simulink model "LPV_Test"  (R2018a)
settings: Solver=VariableStepAuto  StartTime=0.0  StopTime=100  RelTol=1e-3
values from neighbouring files (symbols this model uses):
  A_LPV = [1 0;A_LPV]    [Teste.m]
  B_LPV = [0 0;B_LPV]    [Teste.m]
  R_LPV = [1.2187222 +0.057908761;-2.1510871 +0.29868726;1.0064014 -0.32014911]    [Teste.m]
  S_LPV = [1 0;-0.77614666 -0.086511881;-0.22385334 +0.086511881]    [Teste.m]
  T_LPV = [0.0740365 +0.036446911]    [Teste.m]
  Ts = 0.1    [Teste.m]
settings Model: Creator=marcus  LastModifiedBy=marcus

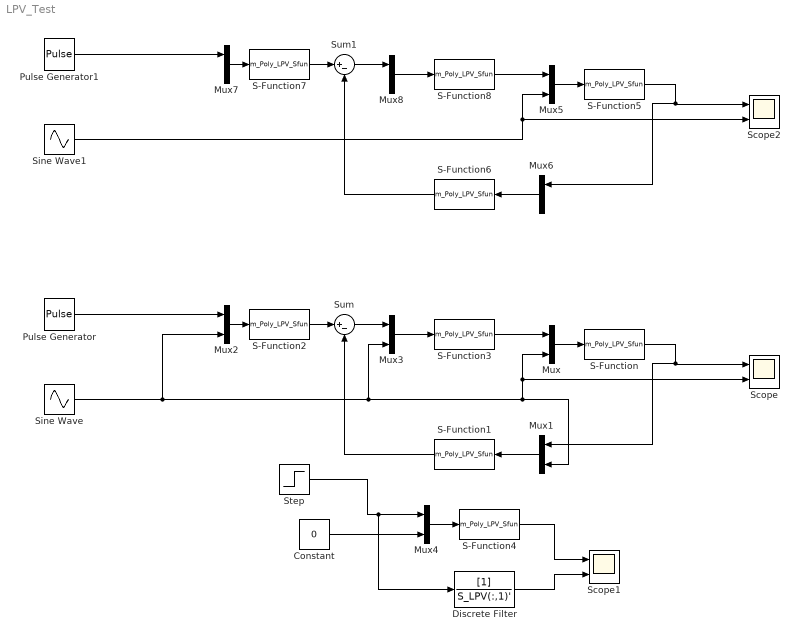
== system LPV_Test ==
  Constant : Constant  Value=0
  Discrete Filter : DiscreteFilter  Denominator=S_LPV(:,1)'
  Mux{,1..8} (9 alike) : Mux  Inputs=2
  Pulse Generator : DiscretePulseGenerator  PulseType=Time based  Period=10  PulseWidth=50
  Pulse Generator1 : DiscretePulseGenerator  PulseType=Time based  Period=10  PulseWidth=50
  S-Function : S-Function  FunctionName=m_Poly_LPV_Sfun  Parameters=Ts,A_LPV,B_LPV  SFunctionDeploymentMode=off  EnableBusSupport=off
  S-Function1 : S-Function  FunctionName=m_Poly_LPV_Sfun  Parameters=Ts,[1 0],R_LPV  SFunctionDeploymentMode=off  EnableBusSupport=off
  S-Function2 : S-Function  FunctionName=m_Poly_LPV_Sfun  Parameters=Ts,[1 0],[T_LPV]  SFunctionDeploymentMode=off  EnableBusSupport=off
  S-Function3 : S-Function  FunctionName=m_Poly_LPV_Sfun  Parameters=Ts,S_LPV,[1 0]  SFunctionDeploymentMode=off  EnableBusSupport=off
  S-Function4 : S-Function  FunctionName=m_Poly_LPV_Sfun  Parameters=Ts,S_LPV,[1 0]  SFunctionDeploymentMode=off  EnableBusSupport=off
  S-Function5 : S-Function  FunctionName=m_Poly_LPV_Sfun  Parameters=Ts,A_LPV,B_LPV  SFunctionDeploymentMode=off  EnableBusSupport=off
  S-Function6 : S-Function  FunctionName=m_Poly_LPV_Sfun  Parameters=Ts,[1 0],R_LPV  SFunctionDeploymentMode=off  EnableBusSupport=off
  S-Function7 : S-Function  FunctionName=m_Poly_LPV_Sfun  Parameters=Ts,[1 0],[T_LPV]  SFunctionDeploymentMode=off  EnableBusSupport=off
  S-Function8 : S-Function  FunctionName=m_Poly_LPV_Sfun  Parameters=Ts,S_LPV,[1 0]  SFunctionDeploymentMode=off  EnableBusSupport=off
  Scope : Scope  NumInputPorts=2
  Scope1 : Scope  NumInputPorts=2
  Scope2 : Scope  NumInputPorts=2
  Sine Wave : Sin  Amplitude=0.4  Bias=0.5  Frequency=0.05  SampleTime=0
  Sine Wave1 : Sin  Amplitude=0.4  Bias=0.5  Frequency=0.05  SampleTime=0
  Step : Step  SampleTime=0
  Sum : Sum  Inputs=|+-
  Sum1 : Sum  Inputs=|+-
  wires:
  Mux/1 -> S-Function/1
  S-Function/1 -> Mux1/1, Scope/1
  Mux2/1 -> S-Function2/1
  Mux1/1 -> S-Function1/1
  Sum/1 -> Mux3/1
  S-Function2/1 -> Sum/1
  Mux3/1 -> S-Function3/1
  Sine Wave/1 -> Mux2/2, Mux1/2, Mux/2, Scope/2, Mux3/2
  S-Function1/1 -> Sum/2
  Pulse Generator/1 -> Mux2/1
  S-Function3/1 -> Mux/1
  Mux4/1 -> S-Function4/1
  Constant/1 -> Mux4/2
  Step/1 -> Discrete Filter/1, Mux4/1
  S-Function4/1 -> Scope1/1
  Discrete Filter/1 -> Scope1/2
  Mux7/1 -> S-Function7/1
  S-Function5/1 -> Mux6/1, Scope2/1
  Mux5/1 -> S-Function5/1
  S-Function7/1 -> Sum1/1
  S-Function6/1 -> Sum1/2
  Mux6/1 -> S-Function6/1
  S-Function8/1 -> Mux5/1
  Sum1/1 -> Mux8/1
  Sine Wave1/1 -> Mux5/2, Scope2/2
  Pulse Generator1/1 -> Mux7/1
  Mux8/1 -> S-Function8/1
